simulink model "close_loop"  (R2022b)
settings: Solver=VariableStepAuto  StartTime=0.0  StopTime=10.0  RelTol=1e-3
undefined symbols (not defined in the file or in its folder): km, Kp, tau
settings Model: Creator=arkad  LastModifiedBy=arkad

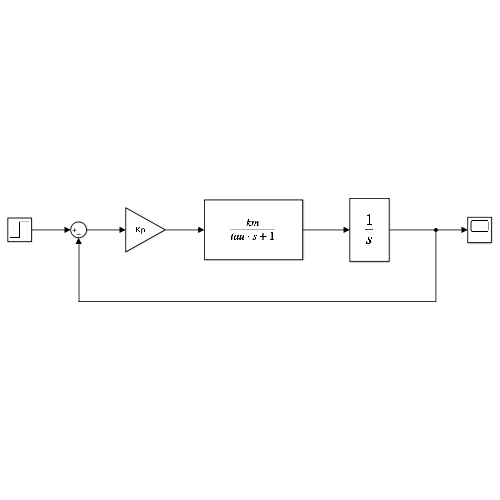
[thumbnail: Simulink's stored preview of the top-level diagram]
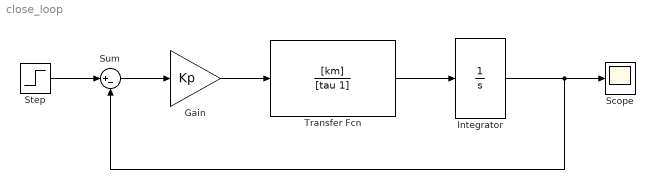
== system close_loop ==
  Gain : Gain  Gain=Kp
  Integrator : Integrator
  Scope : Scope
  Step : Step  SampleTime=0
  Sum : Sum  Inputs=|+-
  Transfer Fcn : TransferFcn  Numerator=[km]  Denominator=[tau 1]
  wires:
  Transfer Fcn/1 -> Integrator/1
  Gain/1 -> Transfer Fcn/1
  Sum/1 -> Gain/1
  Integrator/1 -> Sum/2, Scope/1
  Step/1 -> Sum/1
